simulink model "LAB07_1_copia2"  (R2022b)
settings: Solver=ode8  StartTime=0.0  StopTime=1000  FixedStep=0.1  RelTol=1e-3
values from neighbouring files (symbols this model uses):
  a = 6.843e6    (= 6843000)    [LAB_07_script.m]    (also in LAB_07_with3Dplot.m)
  A0 = eye(3,3)    [LAB_07_script.m]    (also in LAB_07_with3Dplot.m)
  A1 = 0.02    [LAB_07_with3Dplot.m]
  A2 = A1    (= 0.02)    [LAB_07_with3Dplot.m]
  A3 = A1    (= 0.02)    [LAB_07_with3Dplot.m]
  alpha_1 = 0.5    [LAB_07_with3Dplot.m]
  alpha_2 = 0.5    [LAB_07_with3Dplot.m]
  C_d = 2.1    [LAB_07_with3Dplot.m]
  e = 0    [LAB_07_script.m]    (also in LAB_07_with3Dplot.m)
  epsilon = 0.4093    [LAB_07_script.m]    (also in LAB_07_with3Dplot.m)
  G = 6.6743e-11    [LAB_07_script.m]    (also in LAB_07_with3Dplot.m)
  g_01 = -29404.8    [LAB_07_script.m]    (also in LAB_07_with3Dplot.m)
  g_11 = -1450.9    [LAB_07_script.m]    (also in LAB_07_with3Dplot.m)
  h_11 = 4652.5    [LAB_07_script.m]    (also in LAB_07_with3Dplot.m)
  i = 0.1    [LAB_07_script.m]    (also in LAB_07_with3Dplot.m)
  I = 10^-2*diag([100.9,25.1,91.6])    [LAB_07_script.m]    (also in LAB_07_with3Dplot.m)
  j_B = [0.01;0.05;0.01]    [LAB_07_script.m]    (also in LAB_07_with3Dplot.m)
  M_Earth = 5.972e24    (= 5.972e+24)    [LAB_07_script.m]    (also in LAB_07_with3Dplot.m)
  n = sqrt(G*M_Earth/a^3)    [LAB_07_script.m]    (also in LAB_07_with3Dplot.m)
  n_sun = 2*pi/T_sun    (= 1.99238499086e-07)    [LAB_07_script.m]    (also in LAB_07_with3Dplot.m)
  P = F_e/c    (= 4.52666666667e-06)    [LAB_07_script.m]    (also in LAB_07_with3Dplot.m)
  position = 1e-2*[10,0,0;0,10,0;-10,0,0;0,-10,0;0,0,15;                                     0,0,-15;0,45,0;0,45,0;0,-45,0;0,-45,0]    [LAB_07_script.m]    (also in LAB_07_with3Dplot.m)
  R_Earth = 6.378e6    (= 6378000)    [LAB_07_script.m]    (also in LAB_07_with3Dplot.m)
  R_sun = 149597870000    [LAB_07_script.m]    (also in LAB_07_with3Dplot.m)
  rhoD_vector = ones(10,1)*0.1    [LAB_07_script.m]    (also in LAB_07_with3Dplot.m)
  rhoS_vector = ones(10,1)*0.5    [LAB_07_script.m]    (also in LAB_07_with3Dplot.m)
  Surfaces_Matrix = [6e-2;6e-2;6e-2;6e-2;4e-2;4e-2;12e-2;                                                     12e-2;12e-2;12e-2]    [LAB_07_script.m]    (also in LAB_07_with3Dplot.m)
  theta0 = 0    [LAB_07_script.m]    (also in LAB_07_with3Dplot.m)
  Theta_m = deg2rad(11.5)    [LAB_07_script.m]    (also in LAB_07_with3Dplot.m)
  Versor_Surfaces_Matrix = [  1 , 0 ,-1 , 0 , 0 , 0 , 1 ,-1 , 1 ,-1 ... (first row only)    [LAB_07_script.m]    (also in LAB_07_with3Dplot.m)
  w0 = [0;0;0.01]    [LAB_07_script.m]    (also in LAB_07_with3Dplot.m = [1;1;1])
  w_Earth = 7.29e-5    (= 7.29e-05)    [LAB_07_script.m]    (also in LAB_07_with3Dplot.m)
undefined symbols (not defined in the file or in its folder): Gyroscope, HS, magnitude
libraries: simulink_extras x8, matrix_library x5, sharedutil x4, vrlib x3
(part 1 of 2)
settings Model: Creator=ludov  LastModifiedBy=carlorichero

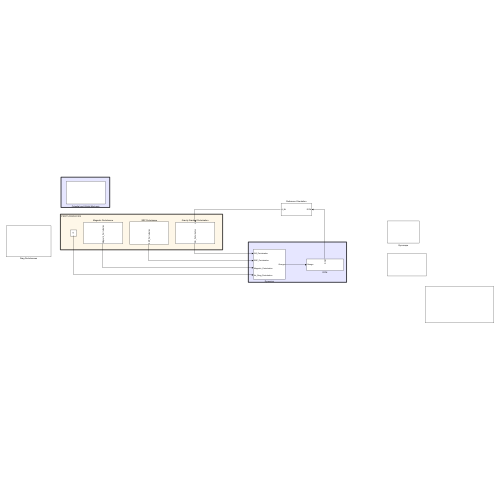
[thumbnail: Simulink's stored preview of the top-level diagram]
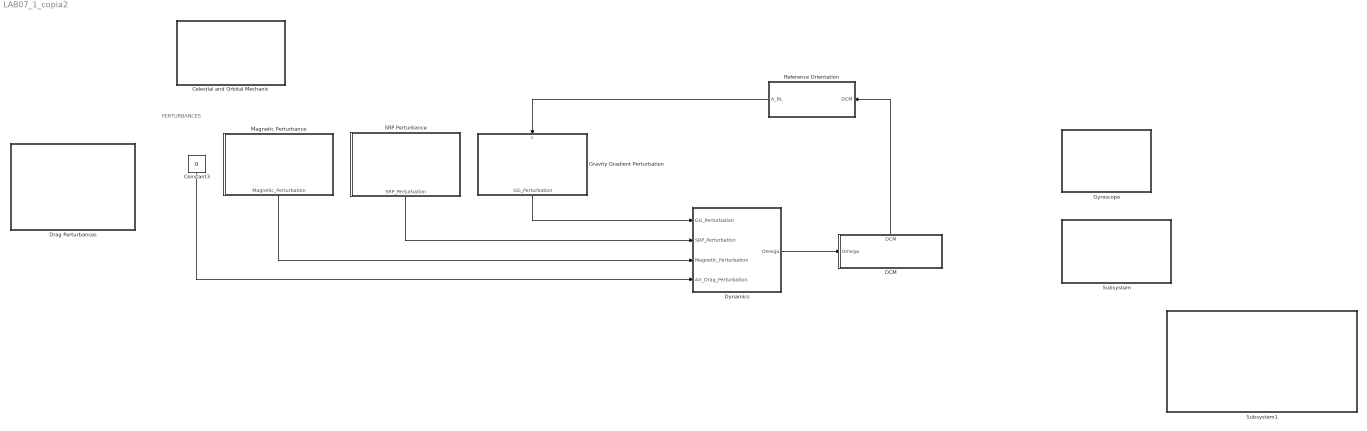
== system LAB07_1_copia2 ==
  note: PERTURBANCES
  " Magnetic Perturbance " : Subsystem
      settings: PortSchema="{\"entries\":[{\"content\":{\"sides\":[{\"content\":{\"connectorIds\":[]},\"type\":\"ConnectorPlacement.EquallySpacedRectSide\",\"uuid\":\"e985e879-37b8-4f0c-a60b-74d5e4b5102c\"},{\"content\":{\"connectorIds\":[],\"side\":\"RIGHT\"},\"type\":\"ConnectorPlacement.EquallySpacedRectSide\",\"uuid\":\"1f0cb419-685e-4dd3-ab14-45869a41b9c2\"},{\"content\":{\"connectorIds\":[],\"side\":\"TOP\"},\"type\":\"ConnectorPlacement.EquallySpacedRectSide\",\"uuid\":\"f8cfa143-02f3-47d6-960d-90021c53ea82\"},{\"content\":{\"connectorIds\":[\"Out1\"],\"side\":\"BOTTOM\"},\"type\":\"ConnectorPlacement.EquallySpacedRectSide\",\"uuid\":\"8ee0ffd0-c547-4f09-8eae-ef027ea96de7\"}]},\"type\":\"ConnectorPlacement.EquallySpacedConnector\",\"uuid\":\"8752746d-e23a-4760-aab6-3f1c0a06bc69\"}],\"packageUris\":[\"http://schema.mathworks.com/mf0/Connector/R2020b\"],\"version\":\"1.0\"}"
  " SRP Perturbance" : Subsystem
      settings: PortSchema="{\"entries\":[{\"content\":{\"sides\":[{\"content\":{\"connectorIds\":[]},\"type\":\"ConnectorPlacement.EquallySpacedRectSide\",\"uuid\":\"e985e879-37b8-4f0c-a60b-74d5e4b5102c\"},{\"content\":{\"connectorIds\":[],\"side\":\"RIGHT\"},\"type\":\"ConnectorPlacement.EquallySpacedRectSide\",\"uuid\":\"1f0cb419-685e-4dd3-ab14-45869a41b9c2\"},{\"content\":{\"connectorIds\":[],\"side\":\"TOP\"},\"type\":\"ConnectorPlacement.EquallySpacedRectSide\",\"uuid\":\"f8cfa143-02f3-47d6-960d-90021c53ea82\"},{\"content\":{\"connectorIds\":[\"Out1\"],\"side\":\"BOTTOM\"},\"type\":\"ConnectorPlacement.EquallySpacedRectSide\",\"uuid\":\"2a12fd6d-c4b7-49e6-8cbf-522d896783f6\"}]},\"type\":\"ConnectorPlacement.EquallySpacedConnector\",\"uuid\":\"8752746d-e23a-4760-aab6-3f1c0a06bc69\"}],\"packageUris\":[\"http://schema.mathworks.com/mf0/Connector/R2020b\"],\"version\":\"1.0\"}"
  Celestial and Orbital Mechanic : Subsystem
  Constant3 : Constant  Value=0
  DCM : Subsystem
      settings: PortSchema="{\"entries\":[{\"content\":{\"sides\":[{\"content\":{\"connectorIds\":[\"In1\"]},\"type\":\"ConnectorPlacement.EquallySpacedRectSide\",\"uuid\":\"36de77ec-8153-48fc-ae5a-ad0b0e2d3ce0\"},{\"content\":{\"connectorIds\":[],\"side\":\"RIGHT\"},\"type\":\"ConnectorPlacement.EquallySpacedRectSide\",\"uuid\":\"5bb36846-76d5-425c-bf3c-97c4283359fa\"},{\"content\":{\"connectorIds\":[\"Out1\"],\"side\":\"TOP\"},\"type\":\"ConnectorPlacement.EquallySpacedRectSide\",\"uuid\":\"8effcbf1-f39c-4e11-8297-2eedf506960c\"}]},\"type\":\"ConnectorPlacement.EquallySpacedConnector\",\"uuid\":\"1130cf8d-ea10-4dfb-b209-46460bb57623\"}],\"packageUris\":[\"http://schema.mathworks.com/mf0/Connector/R2020b\"],\"version\":\"1.0\"}"
  Drag Perturbances : Subsystem
  Dynamics : Subsystem
  Gravity Gradient Perturbation : Subsystem
      settings: PortSchema="{\"entries\":[{\"content\":{\"sides\":[{\"content\":{\"connectorIds\":[]},\"type\":\"ConnectorPlacement.EquallySpacedRectSide\",\"uuid\":\"0f339a99-129b-4972-909e-aa08984290af\"},{\"content\":{\"connectorIds\":[],\"side\":\"RIGHT\"},\"type\":\"ConnectorPlacement.EquallySpacedRectSide\",\"uuid\":\"c349fcfc-19e0-4c37-99ec-428747fba93f\"},{\"content\":{\"connectorIds\":[\"In1\"],\"side\":\"TOP\"},\"type\":\"ConnectorPlacement.EquallySpacedRectSide\",\"uuid\":\"2ac505f4-7a46-421c-9759-99416a32691b\"},{\"content\":{\"connectorIds\":[\"Out1\"],\"side\":\"BOTTOM\"},\"type\":\"ConnectorPlacement.EquallySpacedRectSide\",\"uuid\":\"46063fda-cf86-410f-90fc-74dd4707f3ff\"}]},\"type\":\"ConnectorPlacement.EquallySpacedConnector\",\"uuid\":\"8656328d-f6ad-4baa-a1ea-e4d5445b99d9\"}],\"packageUris\":[\"http://schema.mathworks.com/mf0/Connector/R2020b\"],\"version\":\"1.0\"}"
  Gyroscope : Subsystem
  Reference Orientation : Subsystem
  Subsystem : Subsystem
  Subsystem1 : Subsystem
  wires:
  DCM/1(DCM) -> Reference Orientation/1(DCM)
  Dynamics/1(Omega) -> DCM/1(Omega)
  " SRP Perturbance"/1(SRP_Perturbation) -> Dynamics/2(SRP_Perturbation)
  " Magnetic Perturbance "/1(Magnetic_Perturbation) -> Dynamics/3(Magnetic_Perturbation)
  Constant3/1 -> Dynamics/4(Air_Drag_Perturbation)
  Reference Orientation/1(A_BL) -> Gravity Gradient Perturbation/1(c)
  Gravity Gradient Perturbation/1(GG_Perturbation) -> Dynamics/1(GG_Perturbation)

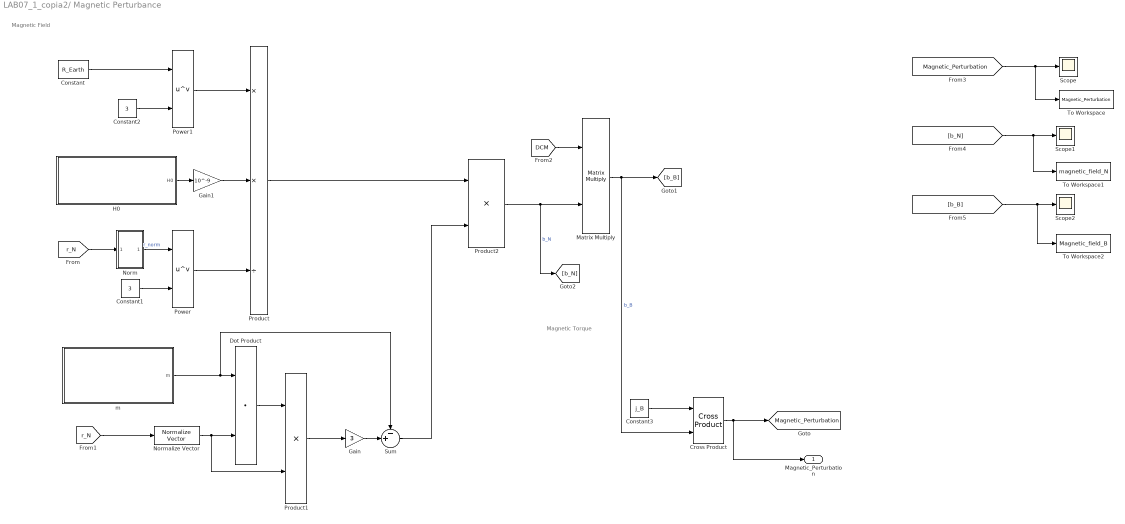
== system LAB07_1_copia2/ Magnetic Perturbance  ==
  note: Magnetic Torque
  note: Magnetic Field
  Constant : Constant  Value=R_Earth
  Constant1 : Constant  Value=3
  Constant2 : Constant  Value=3
  Constant3 : Constant  Value=j_B
  Cross Product : matrix_library/Cross Product
  Dot Product : DotProduct  OutDataTypeStr=Inherit: Inherit via internal rule
  Gain : Gain  Gain=3
  Gain1 : Gain  Gain=10^-9
  H0 : Subsystem
  Matrix Multiply : Product  Multiplication=Matrix(*)
  Norm : Subsystem
  Normalize Vector : vrlib/Utilities/Normalize Vector  maxzero=0
  Power : Math  Operator=pow
  Power1 : Math  Operator=pow
  Product : Product  Inputs=**/
  Product1 : Product
  Product2 : Product
  Scope : Scope
  Scope1 : Scope
  Scope2 : Scope
  Sum : Sum  Inputs=-+|
  To Workspace : ToWorkspace  VariableName=Magnetic_Perturbation  SaveFormat=Timeseries  SampleTime=-1
  To Workspace1 : ToWorkspace  VariableName=magnetic_field_N  SaveFormat=Timeseries  SampleTime=-1
  To Workspace2 : ToWorkspace  VariableName=Magnetic_field_B  SaveFormat=Timeseries  SampleTime=-1
  m : Subsystem
  Magnetic_Perturbation : Outport
  tag scope: Magnetic_Perturbation=global
  wires:
  Constant2/1 -> Power1/2
  Constant/1 -> Power1/1
  Power1/1 -> Product/1
  [r_N] -> Norm/1(In1)
  Constant1/1 -> Power/2
  Norm/1(Out1) -> Power/1  "r_norm"
  Power/1 -> Product/3
  H0/1(H0) -> Gain1/1
  Product/1 -> Product2/1
  m/1(m) -> Dot Product/1, Sum/1
  [r_N] -> Normalize Vector/1
  Normalize Vector/1 -> Product1/2, Dot Product/2
  Gain/1 -> Sum/2
  Dot Product/1 -> Product1/1
  Product1/1 -> Gain/1
  Sum/1 -> Product2/2
  Product2/1 -> [b_N], Matrix Multiply/2  "b_N"
  [DCM] -> Matrix Multiply/1
  Matrix Multiply/1 -> [b_B], Cross Product/2  "b_B"
  Cross Product/1 -> [Magnetic_Perturbation], Magnetic_Perturbation/1
  [Magnetic_Perturbation] -> Scope/1, To Workspace/1
  [b_N] -> To Workspace1/1, Scope1/1
  [b_B] -> To Workspace2/1, Scope2/1
  Gain1/1 -> Product/2
  Constant3/1 -> Cross Product/1

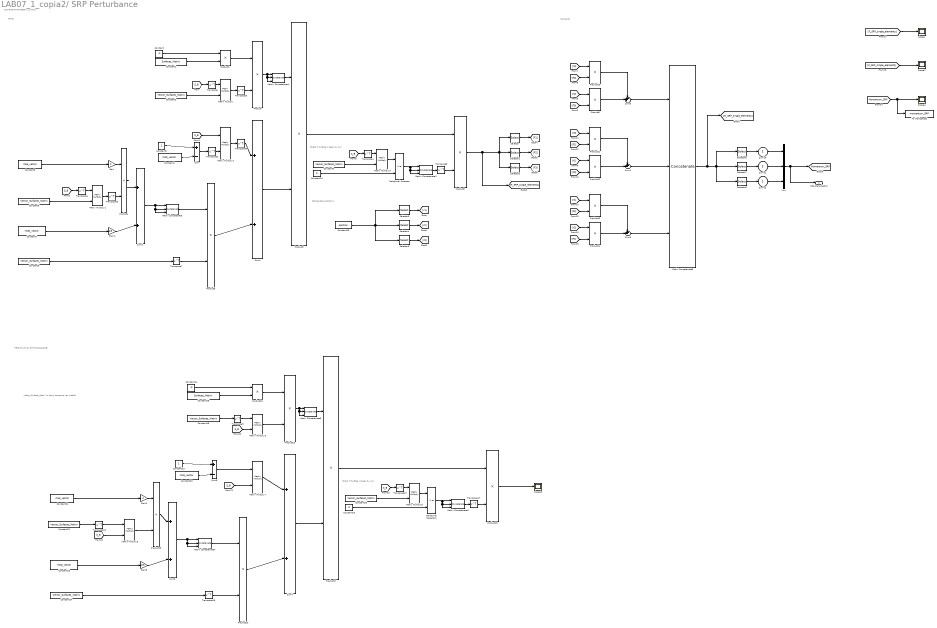
== system LAB07_1_copia2/ SRP Perturbance ==
  note: vector_Surface_Matrix lo devo trasporre nel matlab
  note: TENTATIVO DI OTTIMIZZAZIONE
  note: Moments
  note: Force
  note: Check if surface is seen by sun
  note: SUN RADIATION PERTURBATION
  note: Check if surface is seen by sun
  note: Baricenters positions
  Constant : Constant  Value=-P
  Constant1 : Constant  Value=Surfaces_Matrix
  Constant10 : Constant  Value=0
  Constant13 : Constant  Value=position
  Constant14 : Constant  Value=-P
  Constant15 : Constant  Value=Surfaces_Matrix
  Constant16 : Constant  Value=0
  Constant{2,6,8..9,18,22,24..25} (8 alike) : Constant  Value=Versor_Surfaces_Matrix
  Constant19 : Constant
  Constant{4..5,20..21} (4 alike) : Constant  Value=rhoS_vector
  Constant23 : Constant  Value=rhoD_vector
  Constant3 : Constant
  Constant7 : Constant  Value=rhoD_vector
  Gain : Gain  Gain=2
  Gain1 : Gain  Gain=2/3
  Gain2 : Gain  Gain=2
  Gain3 : Gain  Gain=2/3
  Matrix Concatenate{,1,3..5} (5 alike) : Concatenate  NumInputs=3  Mode=Multidimensional array  ConcatenateDimension=2
  Matrix Concatenate2 : Concatenate  NumInputs=3  Mode=Multidimensional array
  Matrix Concatenate6 : Concatenate  NumInputs=3  Mode=Multidimensional array
  Matrix Multiply{,1..3,5..8} (8 alike) : Product  Multiplication=Matrix(*)
  Mux : Mux  Inputs=3
  Product{,1..5,9..20} (18 alike) : Product
  Relational Operator : RelationalOperator  OutDataTypeStr=boolean  RndMeth=Simplest  InputSameDT=off
  Relational Operator1 : RelationalOperator  OutDataTypeStr=boolean  RndMeth=Simplest  InputSameDT=off
  Scope{,1,3..4} (4 alike) : Scope
  Selector : Selector  NumberOfDimensions=2  InputPortWidth=3  IndexOptions=Select all,Index vector (dialog)  Indices=1,1  OutputSizes=1,1
  Selector1 : Selector  NumberOfDimensions=2  InputPortWidth=3  IndexOptions=Select all,Index vector (dialog)  Indices=1,2  OutputSizes=1,1
  Selector2 : Selector  NumberOfDimensions=2  InputPortWidth=3  IndexOptions=Select all,Index vector (dialog)  Indices=1,3  OutputSizes=1,1
  Selector3 : Selector  NumberOfDimensions=2  InputPortWidth=3  IndexOptions=Select all,Index vector (dialog)  Indices=1,1  OutputSizes=1,1
  Selector4 : Selector  NumberOfDimensions=2  InputPortWidth=3  IndexOptions=Select all,Index vector (dialog)  Indices=1,2  OutputSizes=1,1
  Selector5 : Selector  NumberOfDimensions=2  InputPortWidth=3  IndexOptions=Select all,Index vector (dialog)  Indices=1,3  OutputSizes=1,1
  Selector6 : Selector  NumberOfDimensions=2  InputPortWidth=3  IndexOptions=Select all,Index vector (dialog)  Indices=[1 3],1  OutputSizes=1,1
  Selector7 : Selector  NumberOfDimensions=2  InputPortWidth=3  IndexOptions=Select all,Index vector (dialog)  Indices=[1 3],2  OutputSizes=1,1
  Selector8 : Selector  NumberOfDimensions=2  InputPortWidth=3  IndexOptions=Select all,Index vector (dialog)  Indices=[1 3],3  OutputSizes=1,1
  Sum : Sum  Inputs=+|-
  Sum{1..2,7..8} (4 alike) : Sum  Inputs=+|+
  Sum10 : Sum  Inputs=+
  Sum11 : Sum  Inputs=+
  Sum12 : Sum  Inputs=+
  Sum3 : Sum  Inputs=-+|
  Sum4 : Sum  Inputs=+-|
  Sum5 : Sum  Inputs=+-|
  Sum6 : Sum  Inputs=+|-
  To Workspace1 : ToWorkspace  VariableName=momentum_SRP  SampleTime=-1
  Transpose{,1..10,13,16..17} (14 alike) : Math  Operator=transpose
  SRP_Perturbation : Outport
  tag scope: Momentum_SRP=global
  wires:
  Constant/1 -> Product1/1
  Product1/1 -> Product/1
  Constant1/1 -> Product1/2
  Matrix Multiply/1 -> Transpose5/1
  [S_B] -> Transpose/1
  Constant2/1 -> Matrix Multiply/2
  [S_B] -> Matrix Multiply2/1
  Constant3/1 -> Sum/1
  Constant4/1 -> Sum/2
  Transpose/1 -> Matrix Multiply/1
  Constant5/1 -> Gain/1
  [S_B] -> Transpose1/1
  Constant6/1 -> Matrix Multiply1/2
  Matrix Multiply1/1 -> Transpose3/1
  Gain/1 -> Product4/1
  Constant7/1 -> Gain1/1
  Matrix Multiply2/1 -> Transpose6/1
  Sum/1 -> Transpose2/1
  Transpose2/1 -> Matrix Multiply2/2
  Gain1/1 -> Sum2/2
  Transpose5/1 -> Product/2
  Product4/1 -> Sum2/1
  Transpose1/1 -> Matrix Multiply1/1
  Transpose3/1 -> Product4/2
  Product5/1 -> Sum1/2
  Transpose6/1 -> Sum1/1
  Constant8/1 -> Transpose7/1
  Transpose7/1 -> Product5/2
  Sum2/1 -> Matrix Concatenate/3, Matrix Concatenate/2, Matrix Concatenate/1
  Matrix Concatenate/1 -> Product5/1
  Product/1 -> Matrix Concatenate1/3, Matrix Concatenate1/2, Matrix Concatenate1/1
  Matrix Concatenate1/1 -> Product2/1
  Constant10/1 -> Relational Operator/2
  Sum1/1 -> Product2/2
  [S_B] -> Transpose4/1
  Matrix Multiply3/1 -> Relational Operator/1
  Transpose4/1 -> Matrix Multiply3/1
  Constant9/1 -> Matrix Multiply3/2
  Relational Operator/1 -> Matrix Concatenate2/3, Matrix Concatenate2/2, Matrix Concatenate2/1
  Matrix Concatenate2/1 -> Transpose8/1
  Product2/1 -> Product3/1
  Transpose8/1 -> Product3/2
  Product3/1 -> [F_SRP_single_elements], Selector/1, Selector2/1, Selector1/1
  Constant13/1 -> Selector5/1, Selector4/1, Selector3/1
  Selector3/1 -> [r1]
  Selector4/1 -> [r2]
  Selector5/1 -> [r3]
  Selector/1 -> [F1]
  Selector1/1 -> [F2]
  Selector2/1 -> [F3]
  [r2] -> Product9/1
  [F3] -> Product9/2
  Product9/1 -> Sum3/2
  [F2] -> Product10/2
  [r3] -> Product10/1
  Product10/1 -> Sum3/1
  Product12/1 -> Sum4/2
  [F3] -> Product12/2
  [r1] -> Product12/1
  [r3] -> Product11/1
  [F1] -> Product11/2
  Product11/1 -> Sum4/1
  Product14/1 -> Sum5/2
  [F1] -> Product14/2
  Product13/1 -> Sum5/1
  [r2] -> Product14/1
  [F2] -> Product13/2
  [r1] -> Product13/1
  Sum5/1 -> Matrix Concatenate3/3
  Sum4/1 -> Matrix Concatenate3/2
  Sum3/1 -> Matrix Concatenate3/1
  Matrix Concatenate3/1 -> Selector6/1, Selector7/1, Selector8/1, [M_SRP_single_elements]
  [F_SRP_single_elements] -> Scope/1
  [M_SRP_single_elements] -> Scope1/1
  Matrix Multiply8/1 -> Relational Operator1/1
  Constant18/1 -> Transpose9/1
  Constant15/1 -> Product16/2
  Matrix Multiply6/1 -> Product19/2
  Constant24/1 -> Transpose16/1
  Product18/1 -> Scope3/1
  Sum7/1 -> Product17/2
  Matrix Multiply5/1 -> Product15/2
  Transpose13/1 -> Matrix Multiply8/1
  Product15/1 -> Matrix Concatenate5/3, Matrix Concatenate5/2, Matrix Concatenate5/1
  Constant22/1 -> Transpose10/1
  Relational Operator1/1 -> Matrix Concatenate6/3, Matrix Concatenate6/2, Matrix Concatenate6/1
  Sum8/1 -> Matrix Concatenate4/3, Matrix Concatenate4/2, Matrix Concatenate4/1
  Matrix Concatenate5/1 -> Product17/1
  Transpose17/1 -> Product18/2
  Matrix Concatenate4/1 -> Product20/1
  Matrix Concatenate6/1 -> Transpose17/1
  Matrix Multiply7/1 -> Sum7/1
  Product19/1 -> Sum8/1
  Product20/1 -> Sum7/2
  Constant25/1 -> Matrix Multiply8/2
  Constant20/1 -> Sum6/2
  Gain2/1 -> Product19/1
  [S_B] -> Matrix Multiply6/2
  Constant19/1 -> Sum6/1
  Product16/1 -> Product15/1
  [S_B] -> Transpose13/1
  Product17/1 -> Product18/1
  Transpose16/1 -> Product20/2
  Gain3/1 -> Sum8/2
  Constant21/1 -> Gain2/1
  Constant23/1 -> Gain3/1
  Constant16/1 -> Relational Operator1/2
  Constant14/1 -> Product16/1
  [S_B] -> Matrix Multiply5/2
  [S_B] -> Matrix Multiply7/2
  Sum6/1 -> Matrix Multiply7/1
  Transpose10/1 -> Matrix Multiply6/1
  Transpose9/1 -> Matrix Multiply5/1
  Mux/1 -> [Momentum_SRP], SRP_Perturbation/1
  [Momentum_SRP] -> To Workspace1/1, Scope4/1
  Selector6/1 -> Sum10/1
  Selector7/1 -> Sum11/1
  Selector8/1 -> Sum12/1
  Sum12/1 -> Mux/3
  Sum11/1 -> Mux/2
  Sum10/1 -> Mux/1

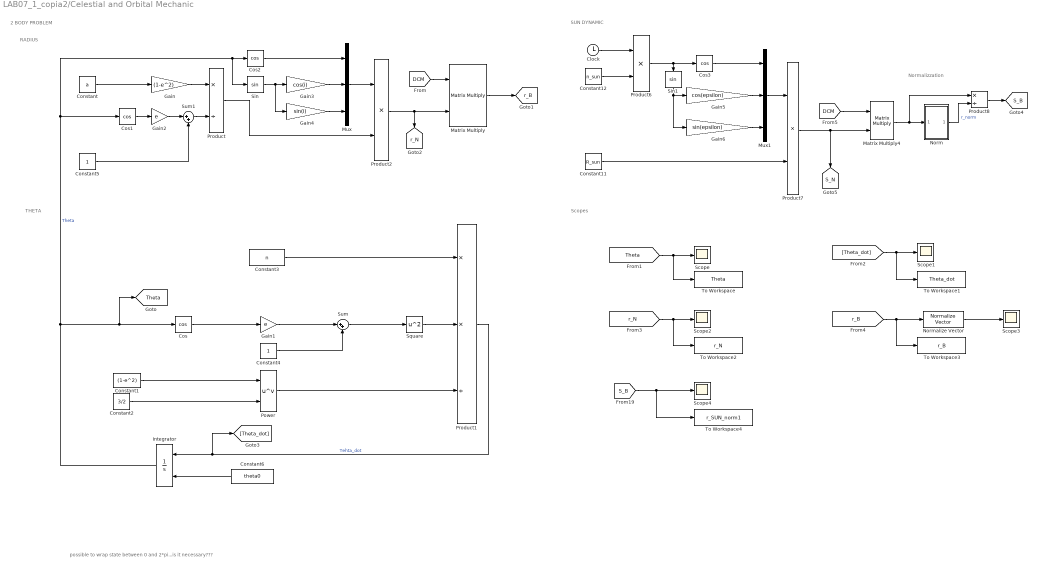
== system LAB07_1_copia2/Celestial and Orbital Mechanic ==
  note: possible to wrap state between 0 and 2*pi...is it necessary???
  note: RADIUS
  note: 2 BODY PROBLEM
  note: THETA
  note: Scopes
  note: Normalizzation
  note: SUN DYNAMIC
  Clock : Clock
  Constant : Constant  Value=a
  Constant1 : Constant  Value=(1-e^2)
  Constant11 : Constant  Value=R_sun
  Constant12 : Constant  Value=n_sun
  Constant2 : Constant  Value=3/2
  Constant3 : Constant  Value=n
  Constant4 : Constant
  Constant5 : Constant
  Constant6 : Constant  Value=theta0
  Cos{,1..3} (4 alike) : Trigonometry  Operator=cos
  Gain : Gain  Gain=(1-e^2)
  Gain1 : Gain  Gain=e
  Gain2 : Gain  Gain=e
  Gain3 : Gain  Gain=cos(i)
  Gain4 : Gain  Gain=sin(i)
  Gain5 : Gain  Gain=cos(epsilon)
  Gain6 : Gain  Gain=sin(epsilon)
  Integrator : Integrator  InitialConditionSource=external  WrappedStateUpperValue=2*pi  WrappedStateLowerValue=0
  Matrix Multiply : Product  Multiplication=Matrix(*)
  Matrix Multiply4 : Product  Multiplication=Matrix(*)
  Mux : Mux  Inputs=3
  Mux1 : Mux  Inputs=3
  Norm : Subsystem
  Normalize Vector : vrlib/Utilities/Normalize Vector  maxzero=0
  Power : Math  Operator=pow
  Product : Product  Inputs=*/
  Product1 : Product  Inputs=**/
  Product2 : Product
  Product6 : Product
  Product7 : Product
  Product8 : Product  Inputs=*/
  Scope{,1..4} (5 alike) : Scope
  Sin : Trigonometry
  Sin1 : Trigonometry
  Square : Math  Operator=square
  Sum : Sum  Inputs=|++
  Sum1 : Sum  Inputs=|++
  To Workspace : ToWorkspace  VariableName=Theta  SaveFormat=Timeseries  SampleTime=-1
  To Workspace1 : ToWorkspace  VariableName=Theta_dot  SaveFormat=Timeseries  SampleTime=-1
  To Workspace2 : ToWorkspace  VariableName=r_N  SampleTime=-1
  To Workspace3 : ToWorkspace  VariableName=r_B  SaveFormat=Timeseries  SampleTime=-1
  To Workspace4 : ToWorkspace  VariableName=r_SUN_norm1  SaveFormat=Timeseries  SampleTime=-1
  tag scope: S_B=global, S_N=global, Theta=global, r_B=global, r_N=global
  wires:
  Constant/1 -> Gain/1
  Gain/1 -> Product/1
  Constant3/1 -> Product1/1
  Cos/1 -> Gain1/1
  Gain1/1 -> Sum/1
  Constant4/1 -> Sum/2
  Sum/1 -> Square/1
  Square/1 -> Product1/2
  Power/1 -> Product1/3
  Constant1/1 -> Power/1
  Constant2/1 -> Power/2
  Product1/1 -> [Theta_dot], Integrator/1  "Tehta_dot"
  Integrator/1 -> Cos2/1, Sin/1, Cos1/1, [Theta], Cos/1  "Theta"
  Cos1/1 -> Gain2/1
  Constant5/1 -> Sum1/2
  Gain2/1 -> Sum1/1
  Sum1/1 -> Product/2
  Constant6/1 -> Integrator/2
  Cos2/1 -> Mux/1
  Sin/1 -> Gain3/1, Gain4/1
  Gain3/1 -> Mux/2
  Gain4/1 -> Mux/3
  Mux/1 -> Product2/1
  Product/1 -> Product2/2
  Product2/1 -> Matrix Multiply/2, [r_N]
  Matrix Multiply/1 -> [r_B]
  [DCM] -> Matrix Multiply/1
  [Theta_dot] -> To Workspace1/1, Scope1/1
  [Theta] -> To Workspace/1, Scope/1
  [r_N] -> To Workspace2/1, Scope2/1
  [r_B] -> To Workspace3/1, Normalize Vector/1
  Clock/1 -> Product6/1
  Sin1/1 -> Gain6/1, Gain5/1
  Constant11/1 -> Product7/2
  Mux1/1 -> Product7/1
  Product6/1 -> Sin1/1, Cos3/1
  Cos3/1 -> Mux1/1
  Norm/1(Out1) -> Product8/2  "r_norm"
  Constant12/1 -> Product6/2
  Gain6/1 -> Mux1/3
  Product7/1 -> [S_N], Matrix Multiply4/2
  Gain5/1 -> Mux1/2
  Product8/1 -> [S_B]
  [DCM] -> Matrix Multiply4/1
  Matrix Multiply4/1 -> Product8/1, Norm/1(In1)
  [S_B] -> To Workspace4/1, Scope4/1
  Normalize Vector/1 -> Scope3/1

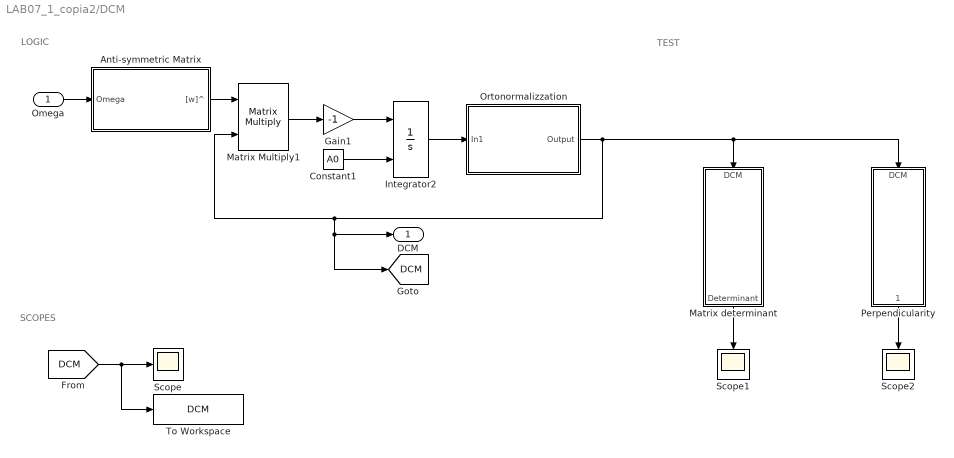
== system LAB07_1_copia2/DCM ==
  note: SCOPES
  note: LOGIC
  note: TEST
  Omega : Inport
  Anti-symmetric Matrix : Subsystem
  Constant1 : Constant  Value=A0
  Gain1 : Gain  Gain=-1
  Integrator2 : Integrator  InitialConditionSource=external
  Matrix Multiply1 : Product  Multiplication=Matrix(*)
  Matrix determinant : Subsystem
  Ortonormalizzation : Subsystem
  Perpendicularity : Subsystem
  Scope : Scope
  Scope1 : Scope
  Scope2 : Scope
  To Workspace : ToWorkspace  VariableName=DCM  SaveFormat=Timeseries  SampleTime=-1
  DCM : Outport
  tag scope: DCM=global
  wires:
  [DCM] -> To Workspace/1, Scope/1
  Anti-symmetric Matrix/1("[w]^") -> Matrix Multiply1/1
  Integrator2/1 -> Ortonormalizzation/1(In1)
  Matrix Multiply1/1 -> Gain1/1
  Ortonormalizzation/1(Output) -> Perpendicularity/1(DCM), Matrix determinant/1(DCM), Matrix Multiply1/2, DCM/1, [DCM]
  Omega/1 -> Anti-symmetric Matrix/1(Omega)
  Gain1/1 -> Integrator2/1
  Constant1/1 -> Integrator2/2
  Matrix determinant/1(Determinant) -> Scope1/1
  Perpendicularity/1(Perpendicularity flag) -> Scope2/1

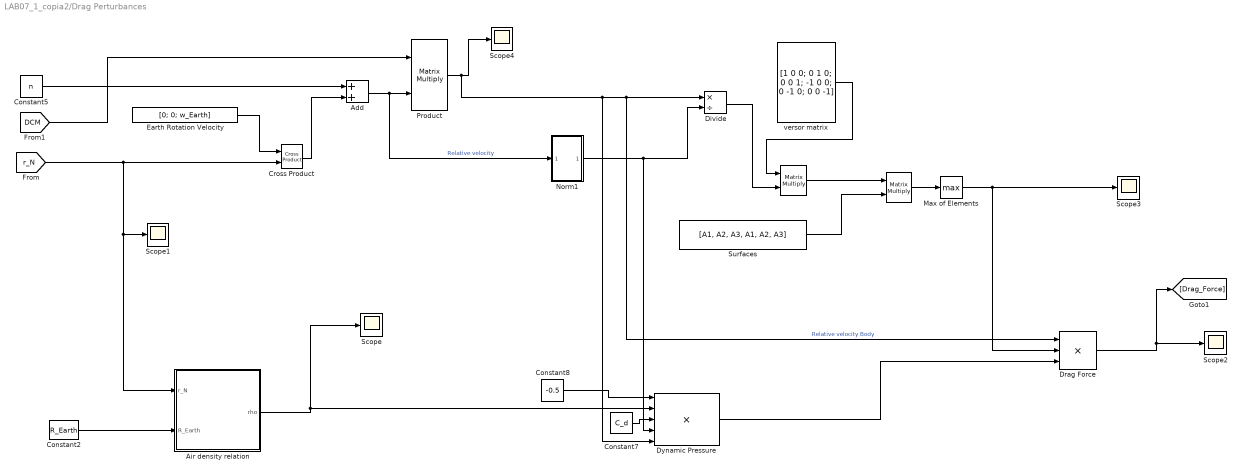
== system LAB07_1_copia2/Drag Perturbances ==
  " " : Product  Multiplication=Matrix(*)
  "   " : Product  Multiplication=Matrix(*)
  Add : Sum
  Air density relation : MATLAB Function  TreatAsAtomicUnit=on
  Constant2 : Constant  Value=R_Earth
  Constant5 : Constant  Value=n
  Constant7 : Constant  Value=C_d
  Constant8 : Constant  Value=-0.5
  Cross Product : vrlib/Utilities/Cross Product
  Divide : Product  Inputs=*/
  Drag Force : Product  Inputs=***
  Dynamic Pressure : Product  Inputs=*****
  Earth Rotation Velocity : Constant  Value=[0; 0; w_Earth]
  Max of Elements : MinMax  Function=max
  Norm1 : Subsystem
  Product : Product  Multiplication=Matrix(*)
  Scope{,1..4} (5 alike) : Scope
  Surfaces : Constant  Value=[A1, A2, A3, A1, A2, A3]
  versor matrix : Constant  Value=[1 0 0; 0 1 0; 0 0 1; -1 0 0; 0 -1 0; 0 0 -1]
  wires:
  [DCM] -> Product/1
  [r_N] -> Scope1/1, Air density relation/1(r_N), Cross Product/2
  Drag Force/1 -> [Drag_Force], Scope2/1
  Constant8/1 -> Dynamic Pressure/1
  Cross Product/1 -> Add/2
  Add/1 -> Norm1/1(In1), Product/2  "Relative velocity"
  Product/1 -> Dynamic Pressure/5, Drag Force/1, Divide/1, Scope4/1  "Relative velocity Body"
  Norm1/1(Out1) -> Dynamic Pressure/4, Divide/2
  Air density relation/1(rho) -> Scope/1, Dynamic Pressure/2
  Earth Rotation Velocity/1 -> Cross Product/1
  Constant5/1 -> Add/1
  " "/1 -> Max of Elements/1
  Max of Elements/1 -> Drag Force/2, Scope3/1
  Dynamic Pressure/1 -> Drag Force/3
  Divide/1 -> "   "/2
  Surfaces/1 -> " "/2
  versor matrix/1 -> "   "/1
  Constant2/1 -> Air density relation/2(R_Earth)
  Constant7/1 -> Dynamic Pressure/3
  "   "/1 -> " "/1

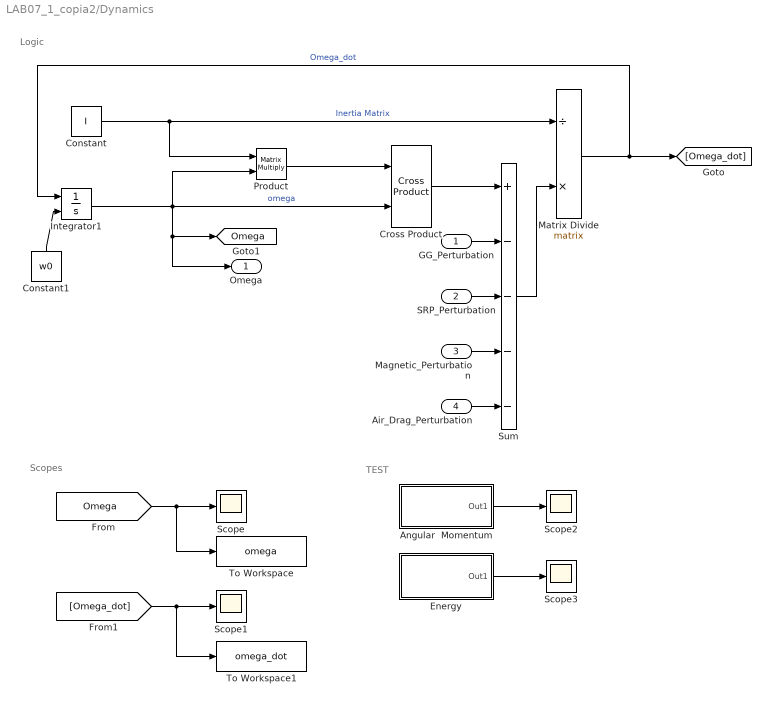
== system LAB07_1_copia2/Dynamics ==
  note: TEST
  note: Logic
  note: Scopes
  GG_Perturbation : Inport
  SRP_Perturbation : Inport  Port=2
  Magnetic_Perturbation : Inport  Port=3
  Air_Drag_Perturbation : Inport  Port=4
  Angular  Momentum : Subsystem
  Constant : Constant  Value=I
  Constant1 : Constant  Value=w0
  Cross Product : matrix_library/Cross Product
  Energy : Subsystem
  Integrator1 : Integrator  InitialConditionSource=external  InitialCondition=w0
  Matrix Divide : Product  Inputs=/*  Multiplication=Matrix(*)
  Product : Product  Multiplication=Matrix(*)
  Scope{,1..3} (4 alike) : Scope
  Sum : Sum  Inputs=+----
  To Workspace : ToWorkspace  VariableName=omega  SaveFormat=Timeseries  SampleTime=-1
  To Workspace1 : ToWorkspace  VariableName=omega_dot  SaveFormat=Timeseries  SampleTime=-1
  Omega : Outport
  tag scope: Omega=global
  wires:
  Product/1 -> Cross Product/1
  Integrator1/1 -> Cross Product/2, Product/2, Omega/1, [Omega]  "omega"
  Matrix Divide/1 -> [Omega_dot], Integrator1/1  "Omega_dot"
  Constant/1 -> Product/1, Matrix Divide/1  "Inertia Matrix"
  [Omega] -> To Workspace/1, Scope/1
  [Omega_dot] -> To Workspace1/1, Scope1/1
  Angular  Momentum/1(Out1) -> Scope2/1
  Energy/1(Out1) -> Scope3/1
  Constant1/1 -> Integrator1/2
  Cross Product/1 -> Sum/1
  Sum/1 -> Matrix Divide/2
  GG_Perturbation/1 -> Sum/2
  Magnetic_Perturbation/1 -> Sum/4
  SRP_Perturbation/1 -> Sum/3
  Air_Drag_Perturbation/1 -> Sum/5

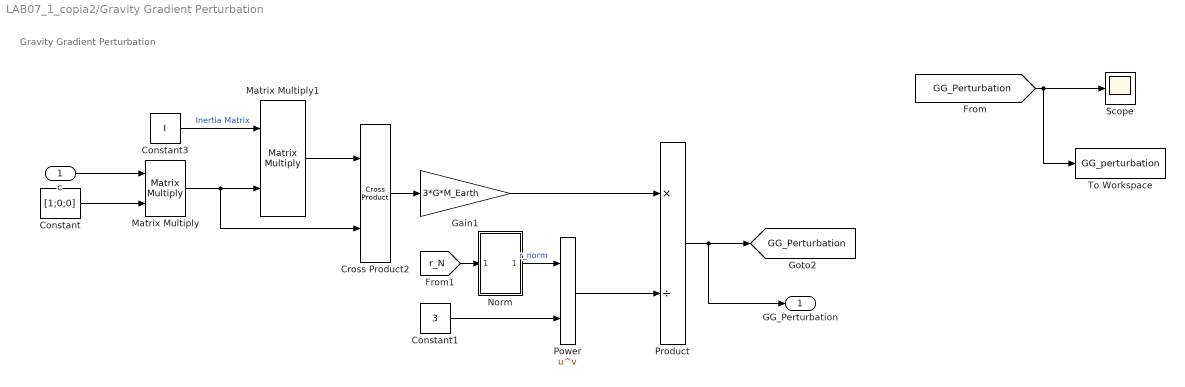
== system LAB07_1_copia2/Gravity Gradient Perturbation ==
  note: Gravity Gradient Perturbation
  c : Inport
  Constant : Constant  Value=[1;0;0]
  Constant1 : Constant  Value=3
  Constant3 : Constant  Value=I
  Cross Product2 : matrix_library/Cross Product
  Gain1 : Gain  Gain=3*G*M_Earth
  Matrix Multiply : Product  Multiplication=Matrix(*)
  Matrix Multiply1 : Product  Multiplication=Matrix(*)
  Norm : Subsystem
  Power : Math  Operator=pow
  Product : Product  Inputs=*/
  Scope : Scope
  To Workspace : ToWorkspace  VariableName=GG_perturbation  SaveFormat=Timeseries  SampleTime=-1
  GG_Perturbation : Outport
  tag scope: GG_Perturbation=global
  wires:
  Constant3/1 -> Matrix Multiply1/1  "Inertia Matrix"
  Matrix Multiply1/1 -> Cross Product2/1
  Cross Product2/1 -> Gain1/1
  [GG_Perturbation] -> Scope/1, To Workspace/1
  Matrix Multiply/1 -> Cross Product2/2, Matrix Multiply1/2
  c/1 -> Matrix Multiply/1
  Constant/1 -> Matrix Multiply/2
  Gain1/1 -> Product/1
  [r_N] -> Norm/1(In1)
  Power/1 -> Product/2
  Product/1 -> [GG_Perturbation], GG_Perturbation/1
  Constant1/1 -> Power/2
  Norm/1(Out1) -> Power/1  "r_norm"

== system LAB07_1_copia2/Gyroscope ==
  Bias : Bias  Bias=Gyroscope.bias_gyro  SaturateOnIntegerOverflow=off
  Constant : Constant  Value=Gyroscope.A_epsilon
  Degrees to Radians : simulink_extras/Transformations/Degrees to Radians
  Gain : Gain  Gain=Gyroscope.Gain
  Matrix Multiply1 : Product  Multiplication=Matrix(*)
  Radians to Degrees : simulink_extras/Transformations/Radians to Degrees
  Scope : Scope
  Scope1 : Scope
  Sum : Sum  Inputs=|++
  White Noise : RandomNumber  Mean=Gyroscope.ARW_mean_value  Variance=0.0001  SampleTime=Gyroscope.sample_time
  Zero-Order Hold : ZeroOrderHold  SampleTime=-1
  wires:
  Gain/1 -> Sum/1
  Sum/1 -> Bias/1
  Bias/1 -> Zero-Order Hold/1
  Zero-Order Hold/1 -> Degrees to Radians/1
  Radians to Degrees/1 -> Gain/1
  Matrix Multiply1/1 -> Radians to Degrees/1, Scope1/1
  White Noise/1 -> Sum/2
  Degrees to Radians/1 -> Scope/1
  Constant/1 -> Matrix Multiply1/1
  [Omega] -> Matrix Multiply1/2

== system LAB07_1_copia2/Reference Orientation ==
  DCM : Inport
  Matrix Multiply : Product  Multiplication=Matrix(*)
  Reference Matrix #1 : Subsystem
  Scope : Scope
  To Workspace : ToWorkspace  VariableName=err  SampleTime=-1
  Transpose : Math  Operator=transpose
  A_BL : Outport
  wires:
  Transpose/1 -> Matrix Multiply/2
  Reference Matrix #1/1(A_LN) -> Transpose/1
  Matrix Multiply/1 -> Scope/1, To Workspace/1, A_BL/1
  DCM/1 -> Matrix Multiply/1

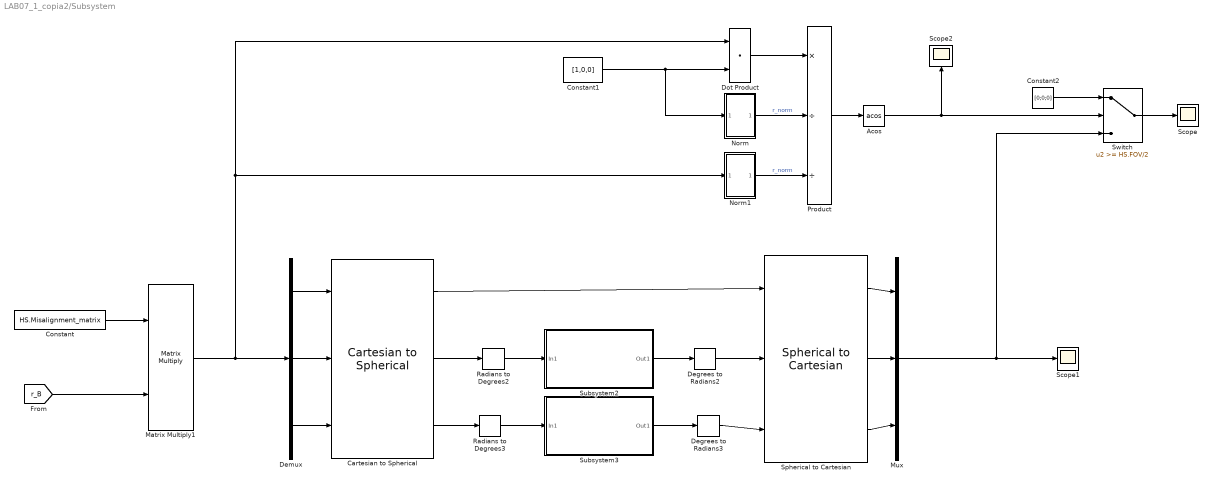
== system LAB07_1_copia2/Subsystem ==
  Acos : Trigonometry  Operator=acos
  Cartesian to Spherical : simulink_extras/Transformations/Cartesian to Spherical
  Constant : Constant  Value=HS.Misalignment_matrix
  Constant1 : Constant  Value=[1,0,0]
  Constant2 : Constant  Value=[0;0;0]
  Degrees to Radians2 : simulink_extras/Transformations/Degrees to Radians
  Degrees to Radians3 : simulink_extras/Transformations/Degrees to Radians
  Demux : Demux  Outputs=3
  Dot Product : DotProduct  OutDataTypeStr=Inherit: Inherit via internal rule
  Matrix Multiply1 : Product  Multiplication=Matrix(*)
  Mux : Mux  Inputs=3
  Norm : Subsystem
  Norm1 : Subsystem
  Product : Product  Inputs=*//
  Radians to Degrees2 : simulink_extras/Transformations/Radians to Degrees
  Radians to Degrees3 : simulink_extras/Transformations/Radians to Degrees
  Scope : Scope
  Scope1 : Scope
  Scope2 : Scope
  Spherical to Cartesian : simulink_extras/Transformations/Spherical to Cartesian
  Subsystem2 : Subsystem
  Subsystem3 : Subsystem
  Switch : Switch  Threshold=HS.FOV/2  SaturateOnIntegerOverflow=off  InputSameDT=off
  wires:
  Constant/1 -> Matrix Multiply1/1
  Constant1/1 -> Dot Product/2, Norm/1(In1)
  Switch/1 -> Scope/1
  Radians to Degrees3/1 -> Subsystem3/1(In1)
  Subsystem3/1(Out1) -> Degrees to Radians3/1
  Subsystem2/1(Out1) -> Degrees to Radians2/1
  Radians to Degrees2/1 -> Subsystem2/1(In1)
  Demux/1 -> Cartesian to Spherical/1
  Demux/2 -> Cartesian to Spherical/2
  Demux/3 -> Cartesian to Spherical/3
  Mux/1 -> Switch/3, Scope1/1
  Cartesian to Spherical/1 -> Spherical to Cartesian/1
  Spherical to Cartesian/3 -> Mux/3
  Spherical to Cartesian/2 -> Mux/2
  Spherical to Cartesian/1 -> Mux/1
  Cartesian to Spherical/2 -> Radians to Degrees2/1
  Degrees to Radians2/1 -> Spherical to Cartesian/2
  Cartesian to Spherical/3 -> Radians to Degrees3/1
  Degrees to Radians3/1 -> Spherical to Cartesian/3
  Matrix Multiply1/1 -> Dot Product/1, Norm1/1(In1), Demux/1
  [r_B] -> Matrix Multiply1/2
  Dot Product/1 -> Product/1
  Norm/1(Out1) -> Product/2  "r_norm"
  Norm1/1(Out1) -> Product/3  "r_norm"
  Product/1 -> Acos/1
  Acos/1 -> Scope2/1, Switch/2
  Constant2/1 -> Switch/1

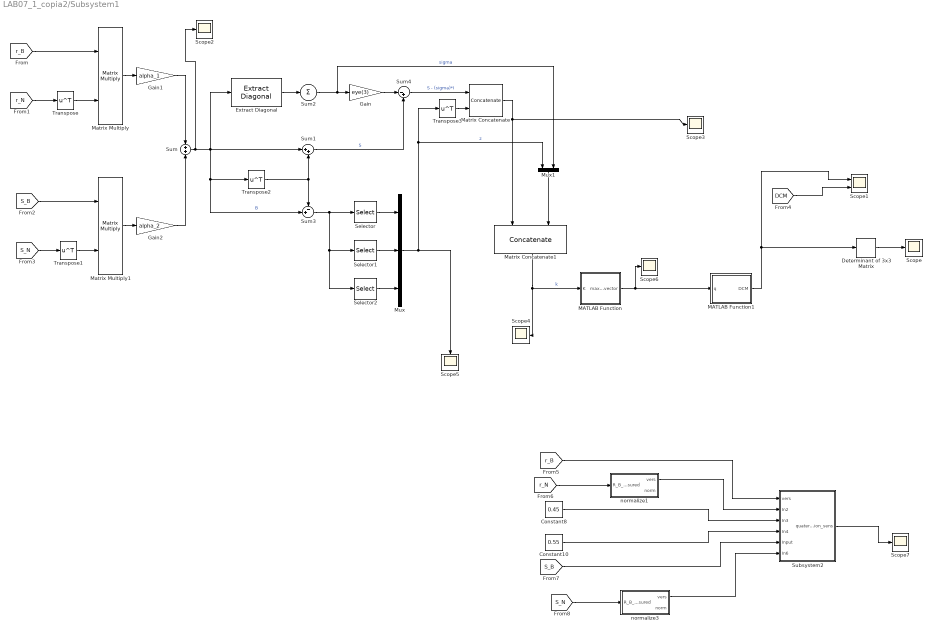
== system LAB07_1_copia2/Subsystem1 ==
  Constant10 : Constant  Value=0.55
  Constant8 : Constant  Value=0.45
  Determinant of 3x3 Matrix : sharedutil/Determinant of 3x3 Matrix  aMode=aMode
      settings: LibrarySourceBlock=|
      | aerolibutil/Determinant of
      | 3x3 Matrix
  Extract Diagonal : matrix_library/Extract Diagonal
      settings: LibrarySourceBlock=|
      | simulink/Matrix
      | Operations/Extract Diagonal
  Gain : Gain  Gain=eye(3)
  Gain1 : Gain  Gain=alpha_1
  Gain2 : Gain  Gain=alpha_2
  MATLAB Function : MATLAB Function  TreatAsAtomicUnit=on
  MATLAB Function1 : MATLAB Function  TreatAsAtomicUnit=on
  Matrix Concatenate : Concatenate  Mode=Multidimensional array
  Matrix Concatenate1 : Concatenate  Mode=Multidimensional array  ConcatenateDimension=2
  Matrix Multiply : Product  Multiplication=Matrix(*)
  Matrix Multiply1 : Product  Multiplication=Matrix(*)
  Mux : Mux  Inputs=3
  Mux1 : Mux  Inputs=2
  Scope{,2..7} (7 alike) : Scope
  Scope1 : Scope  NumInputPorts=2
  Selector : Selector  NumberOfDimensions=2  InputPortWidth=3  IndexOptions=Index vector (dialog),Index vector (dialog)  Indices=2,3  OutputSizes=1,1
  Selector1 : Selector  NumberOfDimensions=2  InputPortWidth=3  IndexOptions=Index vector (dialog),Index vector (dialog)  Indices=3,1  OutputSizes=1,1
  Selector2 : Selector  NumberOfDimensions=2  InputPortWidth=3  IndexOptions=Index vector (dialog),Index vector (dialog)  Indices=1,2  OutputSizes=1,1
  Subsystem2 : Subsystem
  Sum : Sum
  Sum1 : Sum  Inputs=|++
  Sum2 : Sum  Inputs=+
  Sum3 : Sum  Inputs=-+|
  Sum4 : Sum  Inputs=|-+
  Transpose{,1..3} (4 alike) : Math  Operator=transpose
  normalize1 : Subsystem
  normalize3 : Subsystem
  wires:
  [r_B] -> Matrix Multiply/1
  [r_N] -> Transpose/1
  [S_N] -> Transpose1/1
  [S_B] -> Matrix Multiply1/1
  Matrix Multiply/1 -> Gain1/1
  Matrix Multiply1/1 -> Gain2/1
  Transpose/1 -> Matrix Multiply/2
  Transpose1/1 -> Matrix Multiply1/2
  Sum/1 -> Scope2/1, Sum3/2, Transpose2/1, Sum1/1, Extract Diagonal/1  "B"
  Transpose2/1 -> Sum1/2, Sum3/1
  Sum1/1 -> Sum4/2  "S"
  Extract Diagonal/1 -> Sum2/1
  Sum2/1 -> Mux1/2, Gain/1  "sigma"
  Sum3/1 -> Selector2/1, Selector1/1, Selector/1
  Selector2/1 -> Mux/3
  Selector1/1 -> Mux/2
  Selector/1 -> Mux/1
  Mux/1 -> Scope5/1, Transpose3/1, Mux1/1  "z"
  Gain/1 -> Sum4/1
  Sum4/1 -> Matrix Concatenate/1  "S - (sigma)*I"
  Transpose3/1 -> Matrix Concatenate/2
  Matrix Concatenate/1 -> Matrix Concatenate1/1, Scope3/1
  Mux1/1 -> Matrix Concatenate1/2
  Matrix Concatenate1/1 -> Scope4/1, MATLAB Function/1(K)  "k"
  Determinant of 3x3 Matrix/1 -> Scope/1
  [DCM] -> Scope1/2
  Gain1/1 -> Sum/1
  Gain2/1 -> Sum/2
  MATLAB Function1/1(DCM) -> Scope1/1, Determinant of 3x3 Matrix/1
  MATLAB Function/1(max_eigenvector) -> MATLAB Function1/1(q), Scope6/1
  [S_B] -> Subsystem2/5(Input)
  normalize1/1(vers) -> Subsystem2/2(In2)
  [r_B] -> Subsystem2/1(vers)
  Subsystem2/1(quaternion_sens) -> Scope7/1
  Constant8/1 -> Subsystem2/3(In3)
  normalize3/1(vers) -> Subsystem2/6(In6)
  Constant10/1 -> Subsystem2/4(In4)
  [S_N] -> normalize3/1(R_B_measured)
  [r_N] -> normalize1/1(R_B_measured)

== system LAB07_1_copia2/ Magnetic Perturbance /H0 ==
  Constant : Constant  Value=g_01
  Constant1 : Constant  Value=g_11
  Constant2 : Constant  Value=h_11
  Sqrt : Sqrt
  Square : Math  Operator=square
  Square1 : Math  Operator=square
  Square2 : Math  Operator=square
  Sum : Sum  Inputs=+++
  H0 : Outport
  wires:
  Constant/1 -> Square/1
  Constant1/1 -> Square1/1
  Constant2/1 -> Square2/1
  Square/1 -> Sum/1
  Square1/1 -> Sum/2
  Square2/1 -> Sum/3
  Sum/1 -> Sqrt/1
  Sqrt/1 -> H0/1

== system LAB07_1_copia2/ Magnetic Perturbance /Norm ==
  In1 : Inport
  Demux : Demux  Outputs=3
  Square : Math  Operator=square
  Square Root : Sqrt
  Square1 : Math  Operator=square
  Square2 : Math  Operator=square
  Sum : Sum  Inputs=+++
  Out1 : Outport
  wires:
  Demux/3 -> Square2/1
  Sum/1 -> Square Root/1
  Demux/1 -> Square/1
  Square1/1 -> Sum/2
  Demux/2 -> Square1/1
  In1/1 -> Demux/1
  Square2/1 -> Sum/3
  Square/1 -> Sum/1
  Square Root/1 -> Out1/1

== system LAB07_1_copia2/ Magnetic Perturbance /m ==
  Clock : Clock
  Constant : Constant  Value=Theta_m
  Constant1 : Constant  Value=w_Earth
  Cos : Trigonometry  Operator=cos
  Cos1 : Trigonometry  Operator=cos
  Mux : Mux  Inputs=3
  Product : Product
  Product1 : Product
  Product2 : Product
  Sin : Trigonometry
  Sin1 : Trigonometry
  m : Outport
  wires:
  Constant/1 -> Sin/1, Cos1/1
  Clock/1 -> Product/2
  Constant1/1 -> Product/1
  Product/1 -> Sin1/1, Cos/1
  Sin/1 -> Product2/1, Product1/1
  Cos/1 -> Product1/2
  Sin1/1 -> Product2/2
  Product2/1 -> Mux/2
  Product1/1 -> Mux/1
  Mux/1 -> m/1
  Cos1/1 -> Mux/3

== system LAB07_1_copia2/Celestial and Orbital Mechanic/Norm ==
  In1 : Inport
  Demux : Demux  Outputs=3
  Square : Math  Operator=square
  Square Root : Sqrt
  Square1 : Math  Operator=square
  Square2 : Math  Operator=square
  Sum : Sum  Inputs=+++
  Out1 : Outport
  wires:
  Demux/3 -> Square2/1
  Sum/1 -> Square Root/1
  Demux/1 -> Square/1
  Square1/1 -> Sum/2
  Demux/2 -> Square1/1
  In1/1 -> Demux/1
  Square2/1 -> Sum/3
  Square/1 -> Sum/1
  Square Root/1 -> Out1/1

== system LAB07_1_copia2/DCM/Anti-symmetric Matrix ==
  Omega : Inport
  Demux : Demux  Outputs=3
  Gain : Gain  Gain=[0,0,0;0,0,-1;0,1,0]
  Gain1 : Gain  Gain=[0,0,1;0,0,0;-1,0,0]
  Gain2 : Gain  Gain=[0,-1,0;1,0,0;0,0,0]
  Sum : Sum  Inputs=+++
  "[w]^" : Outport
  wires:
  Sum/1 -> "[w]^"/1
  Demux/1 -> Gain/1
  Gain/1 -> Sum/1
  Demux/3 -> Gain2/1
  Gain2/1 -> Sum/3
  Demux/2 -> Gain1/1
  Gain1/1 -> Sum/2
  Omega/1 -> Demux/1

== system LAB07_1_copia2/DCM/Matrix determinant ==
  DCM : Inport
  Determinant of 3x3 Matrix : sharedutil/Determinant of 3x3 Matrix  aMode=aMode
      settings: LibrarySourceBlock=|
      | aerolibutil/Determinant of
      | 3x3 Matrix
  Determinant : Outport
  wires:
  Determinant of 3x3 Matrix/1 -> Determinant/1
  DCM/1 -> Determinant of 3x3 Matrix/1

== system LAB07_1_copia2/DCM/Ortonormalizzation ==
  In1 : Inport
  Gain : Gain  Gain=1.5
  Gain1 : Gain  Gain=0.5
  Matrix Multiply : Product  Inputs=3  Multiplication=Matrix(*)
  Sum : Sum  Inputs=|+-
  Transpose : Math  Operator=transpose
  Output : Outport
  wires:
  Matrix Multiply/1 -> Gain1/1
  Gain/1 -> Sum/1
  In1/1 -> Matrix Multiply/3, Gain/1, Transpose/1, Matrix Multiply/1
  Gain1/1 -> Sum/2
  Transpose/1 -> Matrix Multiply/2
  Sum/1 -> Output/1

== system LAB07_1_copia2/DCM/Perpendicularity ==
  DCM : Inport
  MATLAB Function2 : MATLAB Function  TreatAsAtomicUnit=on
  Perpendicularity flag : Outport
  wires:
  MATLAB Function2/1(perpendicularity_flag) -> Perpendicularity flag/1
  DCM/1 -> MATLAB Function2/1(DCM)

== system LAB07_1_copia2/Drag Perturbances/Norm1 ==
  In1 : Inport
  Demux : Demux  Outputs=3
  Square : Math  Operator=square
  Square Root : Sqrt
  Square1 : Math  Operator=square
  Square2 : Math  Operator=square
  Sum : Sum  Inputs=+++
  Out1 : Outport
  wires:
  Demux/3 -> Square2/1
  Sum/1 -> Square Root/1
  Demux/1 -> Square/1
  Square1/1 -> Sum/2
  Demux/2 -> Square1/1
  In1/1 -> Demux/1
  Square2/1 -> Sum/3
  Square/1 -> Sum/1
  Square Root/1 -> Out1/1

== system LAB07_1_copia2/Dynamics/Angular  Momentum ==
  Constant1 : Constant  Value=I
  Demux : Demux  Outputs=3
  Product1 : Product  Multiplication=Matrix(*)
  Square : Math  Operator=square
  Square Root : Sqrt
  Square1 : Math  Operator=square
  Square2 : Math  Operator=square
  Sum : Sum  Inputs=+++
  Out1 : Outport
  wires:
  [Omega] -> Product1/2
  Constant1/1 -> Product1/1
  Product1/1 -> Demux/1
  Square Root/1 -> Out1/1
  Demux/1 -> Square/1
  Demux/2 -> Square2/1
  Demux/3 -> Square1/1
  Square/1 -> Sum/1
  Square2/1 -> Sum/2
  Square1/1 -> Sum/3
  Sum/1 -> Square Root/1

== system LAB07_1_copia2/Dynamics/Energy ==
  Constant1 : Constant  Value=I
  Gain : Gain  Gain=0.5
  Matrix Multiply : Product  Multiplication=Matrix(*)
  Matrix Multiply1 : Product  Multiplication=Matrix(*)
  Transpose : Math  Operator=transpose
  Out1 : Outport
  wires:
  Matrix Multiply1/1 -> Gain/1
  Matrix Multiply/1 -> Matrix Multiply1/1
  [Omega] -> Matrix Multiply1/2, Transpose/1
  Transpose/1 -> Matrix Multiply/1
  Gain/1 -> Out1/1
  Constant1/1 -> Matrix Multiply/2

== system LAB07_1_copia2/Gravity Gradient Perturbation/Norm ==
  In1 : Inport
  Demux : Demux  Outputs=3
  Square : Math  Operator=square
  Square Root : Sqrt
  Square1 : Math  Operator=square
  Square2 : Math  Operator=square
  Sum : Sum  Inputs=+++
  Out1 : Outport
  wires:
  Demux/3 -> Square2/1
  Sum/1 -> Square Root/1
  Demux/1 -> Square/1
  Square1/1 -> Sum/2
  Demux/2 -> Square1/1
  In1/1 -> Demux/1
  Square2/1 -> Sum/3
  Square/1 -> Sum/1
  Square Root/1 -> Out1/1

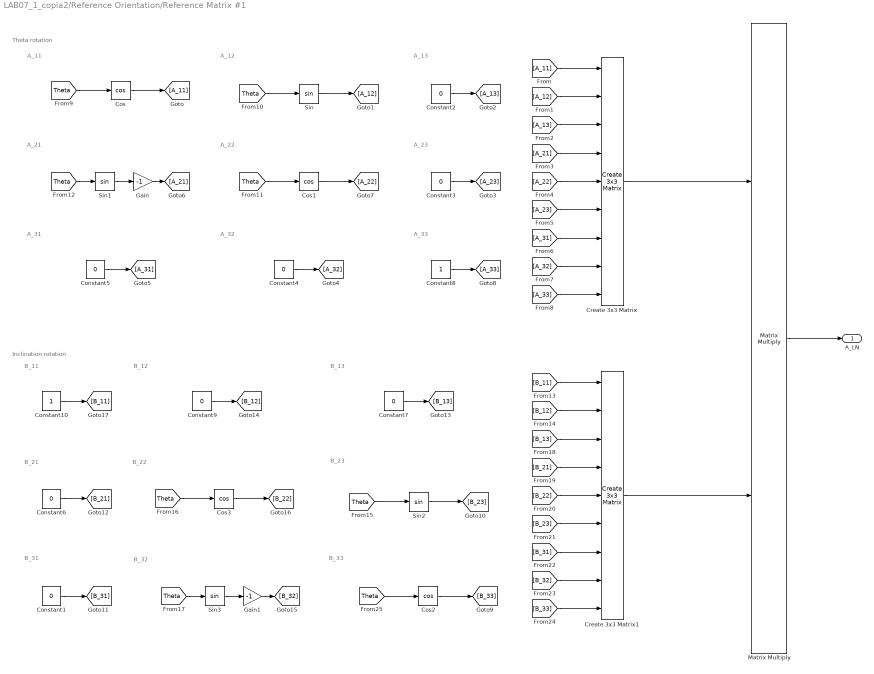
== system LAB07_1_copia2/Reference Orientation/Reference Matrix #1 ==
  note: Theta rotation
  note: A_11
  note: A_12
  note: A_13
  note: A_23
  note: A_33
  note: A_22
  note: A_21
  note: A_31
  note: A_32
  note: B_22
  note: B_33
  note: B_13
  note: B_23
  note: Inclination rotation
  note: B_21
  note: B_32
  note: B_11
  note: B_31
  note: B_12
  Constant{1..7,9} (8 alike) : Constant  Value=0
  Constant10 : Constant
  Constant8 : Constant
  Cos{,1..3} (4 alike) : Trigonometry  Operator=cos
  Create 3x3 Matrix : sharedutil/Create 3x3 Matrix  aMode=aMode
      settings: LibrarySourceBlock=aerolibutil/Create 3x3 Matrix
  Create 3x3 Matrix1 : sharedutil/Create 3x3 Matrix  aMode=aMode
      settings: LibrarySourceBlock=aerolibutil/Create 3x3 Matrix
  Gain : Gain  Gain=-1
  Gain1 : Gain  Gain=-1
  Matrix Multiply : Product  Multiplication=Matrix(*)
  Sin{,1..3} (4 alike) : Trigonometry
  A_LN : Outport
  wires:
  [Theta] -> Cos/1
  Cos/1 -> [A_11]
  Sin/1 -> [A_12]
  Constant2/1 -> [A_13]
  Constant3/1 -> [A_23]
  Constant4/1 -> [A_32]
  Constant5/1 -> [A_31]
  Sin1/1 -> Gain/1
  Cos1/1 -> [A_22]
  Constant8/1 -> [A_33]
  [A_11] -> Create 3x3 Matrix/1
  [A_12] -> Create 3x3 Matrix/2
  [A_13] -> Create 3x3 Matrix/3
  [A_21] -> Create 3x3 Matrix/4
  [A_22] -> Create 3x3 Matrix/5
  [A_23] -> Create 3x3 Matrix/6
  [A_31] -> Create 3x3 Matrix/7
  [A_32] -> Create 3x3 Matrix/8
  [A_33] -> Create 3x3 Matrix/9
  Create 3x3 Matrix/1 -> Matrix Multiply/1
  [Theta] -> Sin/1
  [Theta] -> Cos1/1
  [Theta] -> Sin1/1
  Gain/1 -> [A_21]
  [Theta] -> Cos2/1
  [Theta] -> Sin3/1
  [Theta] -> Cos3/1
  [B_11] -> Create 3x3 Matrix1/1
  Constant6/1 -> [B_21]
  Constant10/1 -> [B_11]
  [B_12] -> Create 3x3 Matrix1/2
  Constant9/1 -> [B_12]
  Sin2/1 -> [B_23]
  Constant7/1 -> [B_13]
  Constant1/1 -> [B_31]
  Cos2/1 -> [B_33]
  Sin3/1 -> Gain1/1
  [B_23] -> Create 3x3 Matrix1/6
  [B_31] -> Create 3x3 Matrix1/7
  [B_33] -> Create 3x3 Matrix1/9
  Cos3/1 -> [B_22]
  Gain1/1 -> [B_32]
  [B_32] -> Create 3x3 Matrix1/8
  Create 3x3 Matrix1/1 -> Matrix Multiply/2
  [B_13] -> Create 3x3 Matrix1/3
  [Theta] -> Sin2/1
  [B_21] -> Create 3x3 Matrix1/4
  [B_22] -> Create 3x3 Matrix1/5
  Matrix Multiply/1 -> A_LN/1

== system LAB07_1_copia2/Subsystem/Norm ==
  In1 : Inport
  Demux : Demux  Outputs=3
  Square : Math  Operator=square
  Square Root : Sqrt
  Square1 : Math  Operator=square
  Square2 : Math  Operator=square
  Sum : Sum  Inputs=+++
  Out1 : Outport
  wires:
  Demux/3 -> Square2/1
  Sum/1 -> Square Root/1
  Demux/1 -> Square/1
  Square1/1 -> Sum/2
  Demux/2 -> Square1/1
  In1/1 -> Demux/1
  Square2/1 -> Sum/3
  Square/1 -> Sum/1
  Square Root/1 -> Out1/1

== system LAB07_1_copia2/Subsystem/Norm1 ==
  In1 : Inport
  Demux : Demux  Outputs=3
  Square : Math  Operator=square
  Square Root : Sqrt
  Square1 : Math  Operator=square
  Square2 : Math  Operator=square
  Sum : Sum  Inputs=+++
  Out1 : Outport
  wires:
  Demux/3 -> Square2/1
  Sum/1 -> Square Root/1
  Demux/1 -> Square/1
  Square1/1 -> Sum/2
  Demux/2 -> Square1/1
  In1/1 -> Demux/1
  Square2/1 -> Sum/3
  Square/1 -> Sum/1
  Square Root/1 -> Out1/1

== system LAB07_1_copia2/Subsystem/Subsystem2 ==
  In1 : Inport
  Abs : Abs  SaturateOnIntegerOverflow=off
  Gain : Gain  Gain=1e-4
  Gain1 : Gain  Gain=1e-4
  Gain2 : Gain  Gain=1e-4
  Square : Math  Operator=square
  Sum : Sum  Inputs=++++
  Out1 : Outport
  wires:
  In1/1 -> Square/1, Abs/1, Gain/1, Sum/1
  Gain/1 -> Sum/2  "Scale"
  Gain1/1 -> Sum/3  "Assimmetry"
  Gain2/1 -> Sum/4  "Non-Linearity"
  Abs/1 -> Gain1/1
  Square/1 -> Gain2/1
  Sum/1 -> Out1/1

== system LAB07_1_copia2/Subsystem/Subsystem3 ==
  In1 : Inport
  Abs : Abs  SaturateOnIntegerOverflow=off
  Gain : Gain  Gain=1e-4
  Gain1 : Gain  Gain=1e-4
  Gain2 : Gain  Gain=1e-4
  Square : Math  Operator=square
  Sum : Sum  Inputs=++++
  Out1 : Outport
  wires:
  In1/1 -> Sum/1, Square/1, Abs/1, Gain/1
  Gain/1 -> Sum/2  "Scale"
  Gain1/1 -> Sum/3  "Assimmetry"
  Gain2/1 -> Sum/4  "Non-Linearity"
  Abs/1 -> Gain1/1
  Square/1 -> Gain2/1
  Sum/1 -> Out1/1

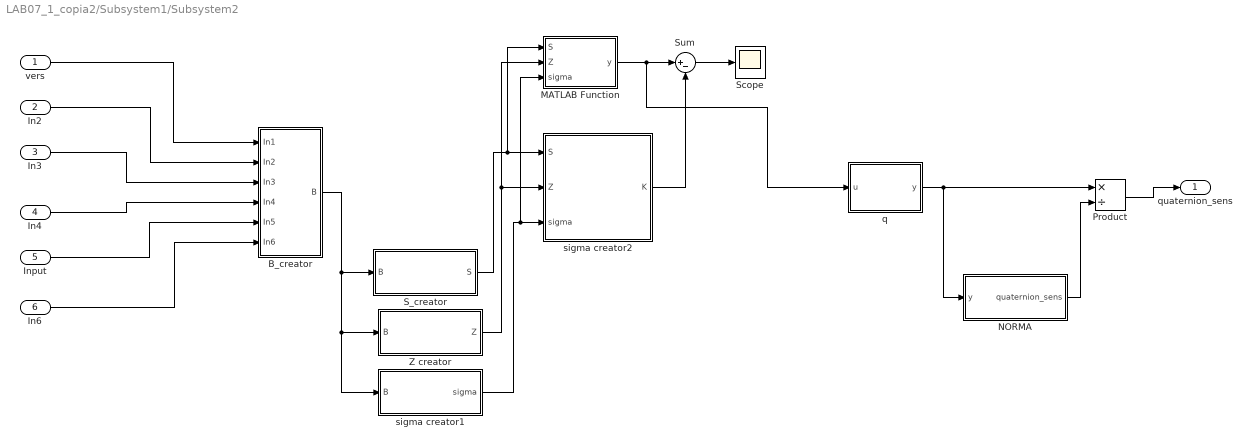
== system LAB07_1_copia2/Subsystem1/Subsystem2 ==
  vers : Inport
  In2 : Inport  Port=2
  In3 : Inport  Port=3
  In4 : Inport  Port=4
  Input : Inport  Port=5
  In6 : Inport  Port=6
  B_creator : Subsystem
  MATLAB Function : MATLAB Function  TreatAsAtomicUnit=on
  NORMA : Subsystem
  Product : Product  Inputs=*/
  S_creator : Subsystem
  Scope : Scope
  Sum : Sum  Inputs=|+-
  Z creator : Subsystem
  q : MATLAB Function  TreatAsAtomicUnit=on
  sigma creator1 : Subsystem
  sigma creator2 : Subsystem
  quaternion_sens : Outport
  wires:
  Z creator/1(Z) -> sigma creator2/2(Z), MATLAB Function/2(Z)
  In3/1 -> B_creator/3(In3)
  In2/1 -> B_creator/2(In2)
  B_creator/1(B) -> S_creator/1(B), sigma creator1/1(B), Z creator/1(B)
  Input/1 -> B_creator/5(In5)
  S_creator/1(S) -> MATLAB Function/1(S), sigma creator2/1(S)
  sigma creator2/1(K) -> Sum/2
  vers/1 -> B_creator/1(In1)
  sigma creator1/1(sigma) -> MATLAB Function/3(sigma), sigma creator2/3(sigma)
  In6/1 -> B_creator/6(In6)
  In4/1 -> B_creator/4(In4)
  q/1(y) -> NORMA/1(y), Product/1
  Product/1 -> quaternion_sens/1
  NORMA/1(quaternion_sens) -> Product/2
  MATLAB Function/1(y) -> q/1(u), Sum/1
  Sum/1 -> Scope/1

== system LAB07_1_copia2/Subsystem1/normalize1 ==
  R_B_measured : Inport
  Demux : Demux  Outputs=3
  Product : Product  Inputs=*/
  Square : Math  Operator=square
  Square Root : Sqrt
  Square1 : Math  Operator=square
  Square2 : Math  Operator=square
  Sum : Sum  Inputs=+++
  vers : Outport
  norm : Outport  Port=2
  wires:
  Product/1 -> vers/1
  Demux/2 -> Square1/1
  R_B_measured/1 -> Demux/1, Product/1
  Sum/1 -> Square Root/1, norm/1
  Demux/1 -> Square/1
  Square1/1 -> Sum/2
  Square/1 -> Sum/1
  Square2/1 -> Sum/3
  Demux/3 -> Square2/1
  Square Root/1 -> Product/2

== system LAB07_1_copia2/Subsystem1/normalize3 ==
  R_B_measured : Inport
  Demux : Demux  Outputs=3
  Product : Product  Inputs=*/
  Square : Math  Operator=square
  Square Root : Sqrt
  Square1 : Math  Operator=square
  Square2 : Math  Operator=square
  Sum : Sum  Inputs=+++
  vers : Outport
  norm : Outport  Port=2
  wires:
  Product/1 -> vers/1
  Demux/2 -> Square1/1
  R_B_measured/1 -> Demux/1, Product/1
  Sum/1 -> Square Root/1, norm/1
  Demux/1 -> Square/1
  Square1/1 -> Sum/2
  Square/1 -> Sum/1
  Square2/1 -> Sum/3
  Demux/3 -> Square2/1
  Square Root/1 -> Product/2

== system LAB07_1_copia2/Subsystem1/Subsystem2/B_creator ==
  In1 : Inport
  In2 : Inport  Port=2
  In3 : Inport  Port=3
  In4 : Inport  Port=4
  In5 : Inport  Port=5
  In6 : Inport  Port=6
  MatrixMultiply : Product  Multiplication=Matrix(*)
  MatrixMultiply2 : Product  Multiplication=Matrix(*)
  Product : Product
  Product1 : Product
  Sum1 : Sum
  Transpose1 : Math  Operator=transpose
  Transpose2 : Math  Operator=transpose
  B : Outport
  wires:
  Product/1 -> Sum1/1
  In2/1 -> Transpose1/1
  Product1/1 -> Sum1/2
  Transpose2/1 -> MatrixMultiply2/2
  MatrixMultiply/1 -> Product/1
  MatrixMultiply2/1 -> Product1/2
  Transpose1/1 -> MatrixMultiply/2
  Sum1/1 -> B/1
  In6/1 -> Transpose2/1
  In4/1 -> Product1/1
  In5/1 -> MatrixMultiply2/1
  In1/1 -> MatrixMultiply/1
  In3/1 -> Product/2

== system LAB07_1_copia2/Subsystem1/Subsystem2/NORMA ==
  y : Inport
  Demux : Demux
  Square{,1..3} (4 alike) : Math  Operator=magnitude^2
  Square Root : Sqrt
  Sum : Sum  Inputs=++++
  quaternion_sens : Outport
  wires:
  y/1 -> Demux/1
  Demux/1 -> Square/1
  Demux/2 -> Square1/1
  Demux/3 -> Square2/1
  Square/1 -> Sum/1
  Square1/1 -> Sum/2
  Square2/1 -> Sum/3
  Sum/1 -> Square Root/1
  Square Root/1 -> quaternion_sens/1
  Demux/4 -> Square3/1
  Square3/1 -> Sum/4

== system LAB07_1_copia2/Subsystem1/Subsystem2/S_creator ==
  B : Inport
  Sum : Sum
  Transpose : Math  Operator=transpose
  S : Outport
  wires:
  B/1 -> Transpose/1, Sum/2
  Transpose/1 -> Sum/1
  Sum/1 -> S/1

== system LAB07_1_copia2/Subsystem1/Subsystem2/Z creator ==
  B : Inport
  Demux : Demux  Outputs=9
  Mux : Mux  Inputs=3
  Reshape : Reshape
  Sum : Sum  Inputs=+-
  Sum1 : Sum  Inputs=+-
  Sum2 : Sum  Inputs=+-
  Z : Outport
  wires:
  B/1 -> Reshape/1
  Reshape/1 -> Demux/1
  Sum/1 -> Mux/1
  Sum1/1 -> Mux/2
  Sum2/1 -> Mux/3
  Demux/8 -> Sum/1
  Demux/6 -> Sum/2
  Demux/3 -> Sum1/1
  Demux/7 -> Sum1/2
  Demux/4 -> Sum2/1
  Demux/2 -> Sum2/2
  Mux/1 -> Z/1

== system LAB07_1_copia2/Subsystem1/Subsystem2/sigma creator1 ==
  B : Inport
  Demux : Demux  Outputs=9
  Extract Diagonal : matrix_library/Extract Diagonal
  Reshape : Reshape
  Sum of Elements : Sum  Inputs=+
  Sum2 : Sum  Inputs=+++
  sigma : Outport
  wires:
  B/1 -> Extract Diagonal/1, Reshape/1
  Reshape/1 -> Demux/1
  Demux/1 -> Sum2/1
  Demux/5 -> Sum2/2
  Demux/9 -> Sum2/3
  Extract Diagonal/1 -> Sum of Elements/1
  Sum of Elements/1 -> sigma/1

== system LAB07_1_copia2/Subsystem1/Subsystem2/sigma creator2 ==
  S : Inport
  Z : Inport  Port=2
  sigma : Inport  Port=3
  Demux : Demux  Outputs=9
  Demux1 : Demux  Outputs=3
  Mux : Mux  Inputs=16
  Reshape : Reshape
  Reshape1 : Reshape  OutputDimensionality=Customize  OutputDimensions=[4,4]
  Sum : Sum  Inputs=+-
  Sum1 : Sum  Inputs=+-
  Sum2 : Sum  Inputs=+-
  K : Outport
  wires:
  Reshape/1 -> Demux/1
  Reshape1/1 -> K/1
  Demux/1 -> Sum/1
  sigma/1 -> Mux/16, Sum2/2, Sum1/2, Sum/2
  Sum/1 -> Mux/1
  Demux/2 -> Mux/2
  Demux/3 -> Mux/3
  Z/1 -> Demux1/1
  Demux1/1 -> Mux/13, Mux/4
  Demux/4 -> Mux/5
  Demux/5 -> Sum1/1
  Sum1/1 -> Mux/6
  Demux/6 -> Mux/7
  Demux1/2 -> Mux/14, Mux/8
  Demux/7 -> Mux/9
  Demux/8 -> Mux/10
  Demux/9 -> Sum2/1
  Sum2/1 -> Mux/11
  Mux/1 -> Reshape1/1
  Demux1/3 -> Mux/15, Mux/12
  S/1 -> Reshape/1

== matlab function LAB07_1_copia2/Subsystem1/MATLAB Function1 ==
  data: q input; DCM output
function DCM = fcn(q)

q1 = q(1);
q2 = q(2);
q3 = q(3);
q4 = q(4);

DCM = [q1^2-q2^2-q3^2+q4^2, 2*(q1*q2+q3*q4), 2*(q1*q3-q2*q4);
        2*(q1*q2-q3*q4), -q1^2+q2^2-q3^2+q4^2, 2*(q2*q3+q1*q4);
        2*(q1*q3+q2*q4), 2*(q2*q3-q1*q4), -q1^2-q2^2+q3^2+q4^2];

end

== matlab function LAB07_1_copia2/Subsystem1/MATLAB Function ==
  data: K input; max_eigenvector output
function max_eigenvector  = eig(K)
[V,D] = eig(K);
[max_eig,linear_index] = max(D(:));
[i, j] = ind2sub(size(K),linear_index); 
max_eigenvector = V(:,j);


end

== matlab function LAB07_1_copia2/Subsystem1/Subsystem2/MATLAB Function ==
  data: S input; y output; Z input; sigma input
function y = fcn(S, Z, sigma)
K=zeros(4,4);
K(1:3,1:3)=S-sigma*eye(3,3);
K(4,1:3)=Z';
K(1:3,4)=Z;
K(4,4)=sigma;
y = K;

== matlab function LAB07_1_copia2/Subsystem1/Subsystem2/q ==
  data: u input; y output
function y = fcn(u)

 
    % Compute eigenvalues and eigenvectors
    [V, D] = eig(u);
    
    % Extract the maximum eigenvalue from the diagonal of D
    [~, idx] = max(diag(D));
    
    % The eigenvector corresponding to the maximum eigenvalue
    v_max = V(:, idx);
    
    y = (V(:,4));

== matlab function LAB07_1_copia2/DCM/Perpendicularity/MATLAB Function2 ==
  data: DCM input; perpendicularity_flag output
function perpendicularity_flag = fcn(DCM)
    

perpendicularity_flag =zeros(3,1);

    x   = DCM(1,:);
    y   = DCM(2,:);
    z   = DCM(3,:);

    perpendicularity_flag(1)=dot(x,y);
    perpendicularity_flag(2)=dot(x,z);
    perpendicularity_flag(3)=dot(z,y);

end
